simulink subsystem "Flux_Eq"  (R2022b)
settings: Solver=VariableStepAuto  StartTime=0.0  StopTime=10.0  RelTol=1e-3
model mask{R=R, Ls=Ls}
  mask prompts: R "Stator Resistance (R)"; Ls "Stator Inductance (Ls)"
settings Model: Creator=MAAM  LastModifiedBy=MAAM

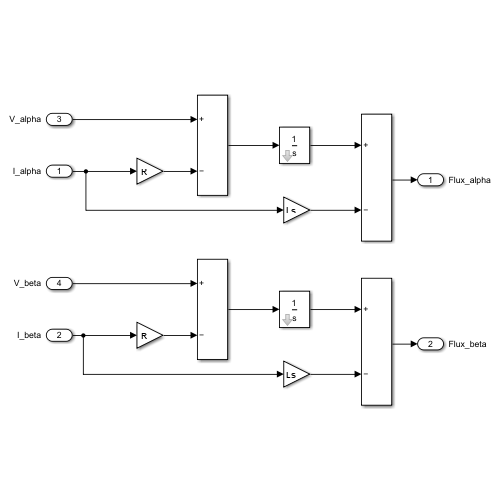
[thumbnail: Simulink's stored preview of the top-level diagram]
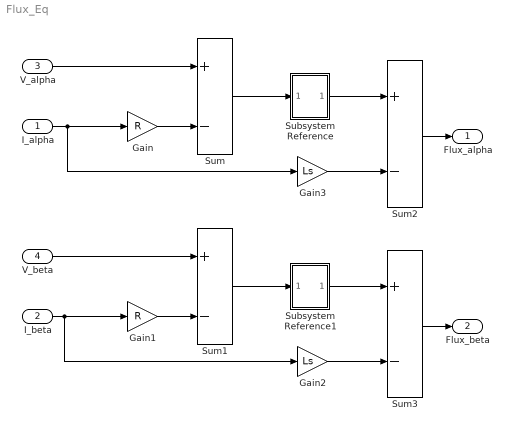
== system Flux_Eq ==
  I_alpha : Inport
  I_beta : Inport  Port=2
  V_alpha : Inport  Port=3
  V_beta : Inport  Port=4
  Gain : Gain  Gain=R
  Gain1 : Gain  Gain=R
  Gain2 : Gain  Gain=Ls
  Gain3 : Gain  Gain=Ls
  Subsystem Reference : Subsystem  ReferencedSubsystem=Integrator  Gain=1.0  Init=0  SampleTime=-1  Ts=0.001
  Subsystem Reference1 : Subsystem  ReferencedSubsystem=Integrator  Gain=1.0  Init=0  SampleTime=-1  Ts=0.001
  Sum{,1..3} (4 alike) : Sum  Inputs=+-
  Flux_alpha : Outport
  Flux_beta : Outport  Port=2
  wires:
  I_alpha/1 -> Gain3/1, Gain/1
  V_alpha/1 -> Sum/1
  Gain/1 -> Sum/2
  Gain1/1 -> Sum1/2
  V_beta/1 -> Sum1/1
  I_beta/1 -> Gain2/1, Gain1/1
  Sum/1 -> Subsystem Reference/1
  Sum1/1 -> Subsystem Reference1/1
  Subsystem Reference/1 -> Sum2/1
  Subsystem Reference1/1 -> Sum3/1
  Sum2/1 -> Flux_alpha/1
  Sum3/1 -> Flux_beta/1
  Gain2/1 -> Sum3/2
  Gain3/1 -> Sum2/2
